simulink model "demapping"  (R2013a)
settings: Solver=VariableStepDiscrete  StartTime=0.0  StopTime=1  RelTol=1e-3
StopFcn:
  | figure(3)
  | hold off
  | plot([-1 1], [0 0],'k:');
  | hold on
  | plot([0 0], [-1 1],'k-');
  | plot([0 x_in_vec(1)], [0 y_in_vec(1)], 'r-','LineWidth',2);
  | plot([0 x_out_vec(1)], [0 y_out_vec(1)],'b-','LineWidth',2);
  | legend('X axis', 'Y axis', 'Input Vector','Output Vector',4);
  | xlabel('X');
  | ylabel('Y');
  | title('Input and Output Vectors');
  | axis([-1 1 -1 1]);
  | axis equal
libraries: xbsIndex_r4 x63
settings Model: Creator=lcrockett  LastModifiedBy=hebin
settings DataIOCC: SignalLoggingSaveFormat=ModelDataLogs
settings OptimizationCC: InlineParams=on  ExpressionDepthLimit=2147483647  InitFltsAndDblsToZero=on
settings DebuggingCC: SaveWithParameterizedLinksMsg=none  FcnCallInpInsideContextMsg=UseLocalSettings  StrictBusMsg=Warning
settings GRTTargetCC: TargetFcnLib=ansi_tfl_tmw.mat  CombineOutputUpdateFcns=off  GRTInterface=on

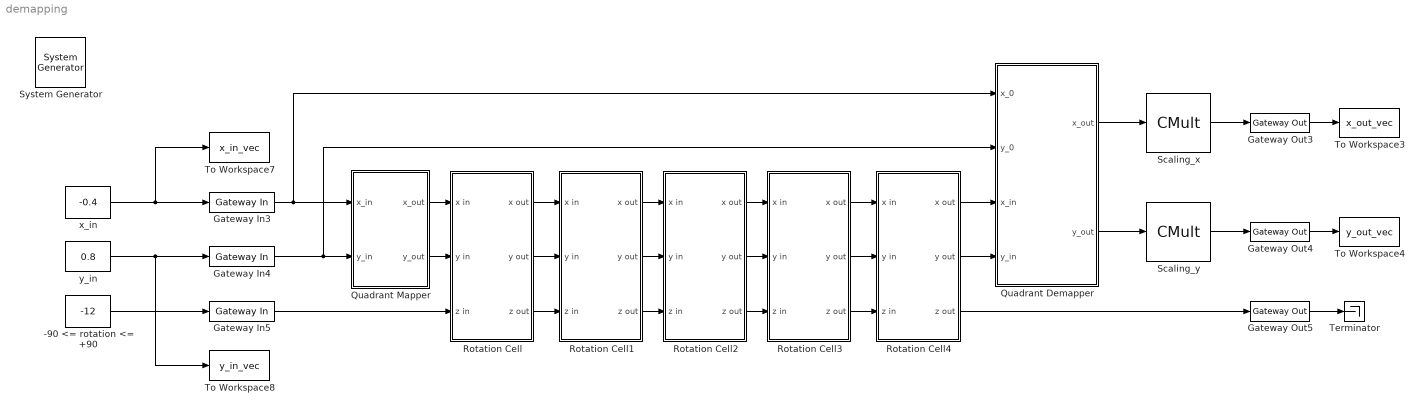
== system demapping ==
  " System Generator" : xbsIndex_r4/ System Generator  Tag=genX  xilinxfamily=virtex2p  part=xc2vp30  speed=-7  package=ff896  synthesis_tool=XST  clock_wrapper=Clock Enables  directory=./netlist  proj_type=Vivado  Synth_file=Vivado Synthesis Defaults  Impl_file=Vivado Implementation Defaults  testbench=off  simulink_period=1  sysclk_period=100  dcm_input_clock_period=100  incr_netlist=off  trim_vbits=Everywhere in SubSystem  dbl_ovrd=According to Block Masks  core_generation=According to Block Masks  run_coregen=off  deprecated_control=off  eval_field=0  block_type=sysgen
      settings: block_version=10.1.2
  -90 <= rotation <= +90 : Constant  Value=-12  SampleTime=1
  Gateway In3 : xbsIndex_r4/Gateway In  gui_display_data_type=Fixed-point  arith_type="Signed  (2's comp)"  n_bits=15  bin_pt=12  preci_type=Single  exp_width=8  frac_width=24  quantization="Round  (unbiased: +/- Inf)"  overflow=Saturate  period=1  UseAsADC=off  ADCChannel='1'  interface=None  automatic_assignment=on  address_offset=hex2dec('00')  intf_description=''  timing_constraint=None  locs_specified=off  LOCs={}  inherit_from_input=off  hdl_port=on  dbl_ovrd=off  io_standard={}  block_type=gatewayin
      settings: infoedit="Gateway in block.  Converts inputs of type Simulink integer, double and fixed point to  Xilinx fixed point type.<P><P>Hardware notes:  In hardware these blocks become top level input ports."  block_version=10.1.2
  Gateway In4 : xbsIndex_r4/Gateway In  gui_display_data_type=Fixed-point  arith_type="Signed  (2's comp)"  n_bits=15  bin_pt=12  preci_type=Single  exp_width=8  frac_width=24  quantization="Round  (unbiased: +/- Inf)"  overflow=Saturate  period=1  UseAsADC=off  ADCChannel='1'  interface=None  automatic_assignment=on  address_offset=hex2dec('00')  intf_description=''  timing_constraint=None  locs_specified=off  LOCs={}  inherit_from_input=off  hdl_port=on  dbl_ovrd=off  io_standard={}  block_type=gatewayin
      settings: infoedit="Gateway in block.  Converts inputs of type Simulink integer, double and fixed point to  Xilinx fixed point type.<P><P>Hardware notes:  In hardware these blocks become top level input ports."  block_version=10.1.2
  Gateway In5 : xbsIndex_r4/Gateway In  gui_display_data_type=Fixed-point  arith_type="Signed  (2's comp)"  n_bits=20  bin_pt=12  preci_type=Single  exp_width=8  frac_width=24  quantization="Round  (unbiased: +/- Inf)"  overflow=Saturate  period=1  UseAsADC=off  ADCChannel='1'  interface=None  automatic_assignment=on  address_offset=hex2dec('00')  intf_description=''  timing_constraint=None  locs_specified=off  LOCs={}  inherit_from_input=off  hdl_port=on  dbl_ovrd=off  io_standard={}  block_type=gatewayin
      settings: infoedit="Gateway in block.  Converts inputs of type Simulink integer, double and fixed point to  Xilinx fixed point type.<P><P>Hardware notes:  In hardware these blocks become top level input ports."  block_version=10.1.2
  Gateway Out3 : xbsIndex_r4/Gateway Out  inherit_from_input=off  hdl_port=on  rows=1  columns=1  UseAsDAC=off  DACChannel='1'  interface=None  automatic_assignment=on  address_offset=hex2dec('00')  intf_description=''  timing_constraint=None  locs_specified=off  LOCs={}  io_standard={}  block_type=gatewayout
      settings: infoedit="Gateway out block.  Converts Xilinx fixed point inputs into ouputs of type Simulink integer, double, or fixed point.<P><P>Hardware notes:  In hardware these blocks become top level output ports or are discarded, depending on how they are configured."  block_version=10.1.2
  Gateway Out4 : xbsIndex_r4/Gateway Out  inherit_from_input=off  hdl_port=on  rows=1  columns=1  UseAsDAC=off  DACChannel='1'  interface=None  automatic_assignment=on  address_offset=hex2dec('00')  intf_description=''  timing_constraint=None  locs_specified=off  LOCs={}  io_standard={}  block_type=gatewayout
      settings: infoedit="Gateway out block.  Converts Xilinx fixed point inputs into ouputs of type Simulink integer, double, or fixed point.<P><P>Hardware notes:  In hardware these blocks become top level output ports or are discarded, depending on how they are configured."  block_version=10.1.2
  Gateway Out5 : xbsIndex_r4/Gateway Out  inherit_from_input=off  hdl_port=on  rows=1  columns=1  UseAsDAC=off  DACChannel='1'  interface=None  automatic_assignment=on  address_offset=hex2dec('00')  intf_description=''  timing_constraint=None  locs_specified=off  LOCs={}  io_standard={}  block_type=gatewayout
      settings: infoedit="Gateway out block.  Converts Xilinx fixed point inputs into ouputs of type Simulink integer, double, or fixed point.<P><P>Hardware notes:  In hardware these blocks become top level output ports or are discarded, depending on how they are configured."  block_version=10.1.2
  Quadrant Demapper : Subsystem
  Quadrant Mapper : Subsystem
  Rotation Cell : Subsystem  mask(Rotation Cell){i=0}
      mask prompts: i "Number of Iterations (i)"
  Rotation Cell1 : Subsystem  mask(Rotation Cell){i=1}
      mask prompts: i "Number of Iterations (i)"
  Rotation Cell2 : Subsystem  mask(Rotation Cell){i=2}
      mask prompts: i "Number of Iterations (i)"
  Rotation Cell3 : Subsystem  mask(Rotation Cell){i=3}
      mask prompts: i "Number of Iterations (i)"
  Rotation Cell4 : Subsystem  mask(Rotation Cell){i=4}
      mask prompts: i "Number of Iterations (i)"
  Scaling_x : xbsIndex_r4/CMult  const=0.607648256256168  gui_display_data_type=Fixed-point  const_n_bits=15  const_bin_pt=12  float_type=Single  exp_bits=8  fraction_bits=24  en=off  latency=0  precision=User Defined  arith_type="Signed  (2's comp)"  n_bits=15  bin_pt=12  quantization=Truncate  overflow=Wrap  use_behavioral_HDL=off  mem_type=Distributed RAM  pipeline=off  use_rpm=off  placement_style=Rectangular Shape  dbl_ovrd=off  block_type=cmult
      settings: block_version=10.1.2
  Scaling_y : xbsIndex_r4/CMult  const=0.607648256256168  gui_display_data_type=Fixed-point  const_n_bits=15  const_bin_pt=12  float_type=Single  exp_bits=8  fraction_bits=24  en=off  latency=0  precision=User Defined  arith_type="Signed  (2's comp)"  n_bits=15  bin_pt=12  quantization=Truncate  overflow=Wrap  use_behavioral_HDL=off  mem_type=Distributed RAM  pipeline=off  use_rpm=off  placement_style=Rectangular Shape  dbl_ovrd=off  block_type=cmult
      settings: block_version=10.1.2
  Terminator : Terminator
  To Workspace3 : ToWorkspace  VariableName=x_out_vec  SampleTime=-1
  To Workspace4 : ToWorkspace  VariableName=y_out_vec  SampleTime=-1
  To Workspace7 : ToWorkspace  VariableName=x_in_vec  SampleTime=-1
  To Workspace8 : ToWorkspace  VariableName=y_in_vec  SampleTime=-1
  x_in : Constant  Value=-0.4  SampleTime=1
  y_in : Constant  Value=0.8  SampleTime=1
  wires:
  Gateway In5/1 -> Rotation Cell/3(z in)
  -90 <= rotation <= +90/1 -> Gateway In5/1
  x_in/1 -> Gateway In3/1, To Workspace7/1
  y_in/1 -> To Workspace8/1, Gateway In4/1
  Gateway Out3/1 -> To Workspace3/1
  Gateway Out4/1 -> To Workspace4/1
  Gateway Out5/1 -> Terminator/1
  Gateway In3/1 -> Quadrant Mapper/1(x_in), Quadrant Demapper/1(x_0)
  Quadrant Mapper/1(x_out) -> Rotation Cell/1(x in)
  Gateway In4/1 -> Quadrant Mapper/2(y_in), Quadrant Demapper/2(y_0)
  Quadrant Mapper/2(y_out) -> Rotation Cell/2(y in)
  Rotation Cell/1(x out) -> Rotation Cell1/1(x in)
  Rotation Cell/2(y out) -> Rotation Cell1/2(y in)
  Rotation Cell/3(z out) -> Rotation Cell1/3(z in)
  Rotation Cell1/1(x out) -> Rotation Cell2/1(x in)
  Rotation Cell1/2(y out) -> Rotation Cell2/2(y in)
  Rotation Cell1/3(z out) -> Rotation Cell2/3(z in)
  Rotation Cell2/1(x out) -> Rotation Cell3/1(x in)
  Rotation Cell2/2(y out) -> Rotation Cell3/2(y in)
  Rotation Cell2/3(z out) -> Rotation Cell3/3(z in)
  Rotation Cell3/1(x out) -> Rotation Cell4/1(x in)
  Rotation Cell3/2(y out) -> Rotation Cell4/2(y in)
  Rotation Cell3/3(z out) -> Rotation Cell4/3(z in)
  Scaling_x/1 -> Gateway Out3/1
  Rotation Cell4/3(z out) -> Gateway Out5/1
  Rotation Cell4/2(y out) -> Quadrant Demapper/4(y_in)
  Rotation Cell4/1(x out) -> Quadrant Demapper/3(x_in)
  Quadrant Demapper/1(x_out) -> Scaling_x/1
  Quadrant Demapper/2(y_out) -> Scaling_y/1
  Scaling_y/1 -> Gateway Out4/1

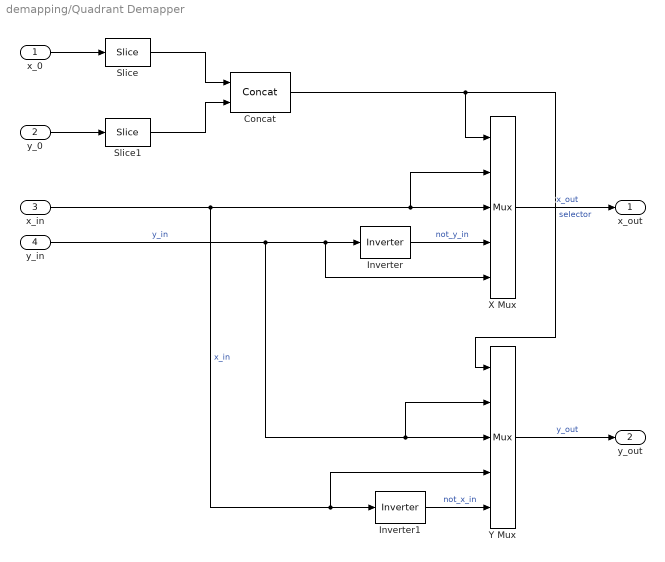
== system demapping/Quadrant Demapper ==
  x_0 : Inport
  y_0 : Inport  Port=2
  x_in : Inport  Port=3
  y_in : Inport  Port=4
  Concat : xbsIndex_r4/Concat  num_inputs=2  dbl_ovrd=off  block_type=concat
      settings: block_version=10.1.2
  Inverter : xbsIndex_r4/Inverter  en=off  latency=0  dbl_ovrd=off  block_type=inv
      settings: block_version=10.1.2
  Inverter1 : xbsIndex_r4/Inverter  en=off  latency=0  dbl_ovrd=off  block_type=inv
      settings: block_version=10.1.2
  Slice : xbsIndex_r4/Slice  nbits=1  boolean_output=on  mode=Upper Bit Location + Width  bit1=0  base1=MSB of Input  bit0=0  base0=LSB of Input  dbl_ovrd=off  block_type=slice
      settings: infoedit="Extracts a given range of bits from each input sample and presents it at the output.  The output type is ordinarily unsigned with binary point at zero, but can be Boolean when the slice is one bit wide.<P><P>Hardware notes: In hardware this block costs nothing."  block_version=VER_STRING_GOES_HERE
  Slice1 : xbsIndex_r4/Slice  nbits=1  boolean_output=on  mode=Upper Bit Location + Width  bit1=0  base1=MSB of Input  bit0=0  base0=LSB of Input  dbl_ovrd=off  block_type=slice
      settings: infoedit="Extracts a given range of bits from each input sample and presents it at the output.  The output type is ordinarily unsigned with binary point at zero, but can be Boolean when the slice is one bit wide.<P><P>Hardware notes: In hardware this block costs nothing."  block_version=VER_STRING_GOES_HERE
  X Mux : xbsIndex_r4/Mux  inputs=4  en=off  latency=0  precision=User Defined  arith_type="Signed  (2's comp)"  n_bits=16  bin_pt=14  quantization=Truncate  overflow=Wrap  dbl_ovrd=off  block_type=mux
      settings: xl_area=[0, 0, 0, 0, 0, 0, 0]  block_version=VER_STRING_GOES_HERE
  Y Mux : xbsIndex_r4/Mux  inputs=4  en=off  latency=0  precision=User Defined  arith_type="Signed  (2's comp)"  n_bits=16  bin_pt=14  quantization=Truncate  overflow=Wrap  dbl_ovrd=off  block_type=mux
      settings: xl_area=[0, 0, 0, 0, 0, 0, 0]  block_version=VER_STRING_GOES_HERE
  x_out : Outport
  y_out : Outport  Port=2
  wires:
  Slice/1 -> Concat/1
  Slice1/1 -> Concat/2
  Concat/1 -> X Mux/1, Y Mux/1  "selector"
  y_0/1 -> Slice1/1
  X Mux/1 -> x_out/1  "x_out"
  Y Mux/1 -> y_out/1  "y_out"
  x_0/1 -> Slice/1
  x_in/1 -> X Mux/2, X Mux/3, Inverter1/1, Y Mux/4  "x_in"
  y_in/1 -> X Mux/5, Inverter/1, Y Mux/3, Y Mux/2  "y_in"
  Inverter/1 -> X Mux/4  "not_y_in"
  Inverter1/1 -> Y Mux/5  "not_x_in"

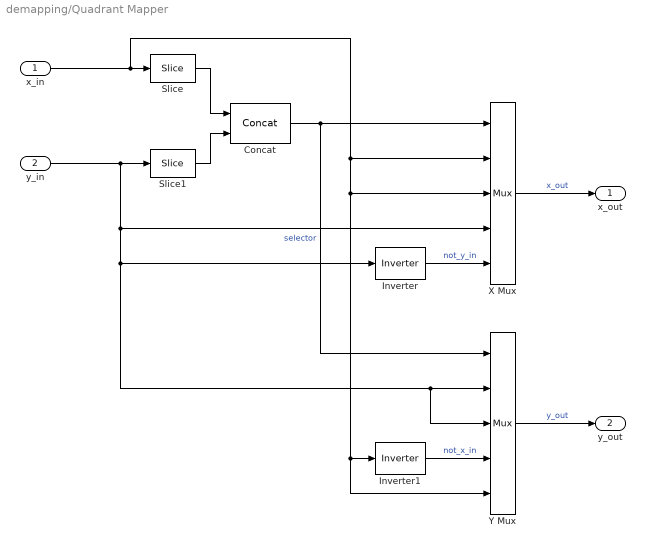
== system demapping/Quadrant Mapper ==
  x_in : Inport
  y_in : Inport  Port=2
  Concat : xbsIndex_r4/Concat  num_inputs=2  dbl_ovrd=off  block_type=concat
      settings: block_version=10.1.2
  Inverter : xbsIndex_r4/Inverter  en=off  latency=0  dbl_ovrd=off  block_type=inv
      settings: block_version=10.1.2
  Inverter1 : xbsIndex_r4/Inverter  en=off  latency=0  dbl_ovrd=off  block_type=inv
      settings: block_version=10.1.2
  Slice : xbsIndex_r4/Slice  nbits=1  boolean_output=on  mode=Upper Bit Location + Width  bit1=0  base1=MSB of Input  bit0=0  base0=LSB of Input  dbl_ovrd=off  block_type=slice
      settings: infoedit="Extracts a given range of bits from each input sample and presents it at the output.  The output type is ordinarily unsigned with binary point at zero, but can be Boolean when the slice is one bit wide.<P><P>Hardware notes: In hardware this block costs nothing."  block_version=VER_STRING_GOES_HERE
  Slice1 : xbsIndex_r4/Slice  nbits=1  boolean_output=on  mode=Upper Bit Location + Width  bit1=0  base1=MSB of Input  bit0=0  base0=LSB of Input  dbl_ovrd=off  block_type=slice
      settings: infoedit="Extracts a given range of bits from each input sample and presents it at the output.  The output type is ordinarily unsigned with binary point at zero, but can be Boolean when the slice is one bit wide.<P><P>Hardware notes: In hardware this block costs nothing."  block_version=VER_STRING_GOES_HERE
  X Mux : xbsIndex_r4/Mux  inputs=4  en=off  latency=0  precision=User Defined  arith_type="Signed  (2's comp)"  n_bits=16  bin_pt=14  quantization=Truncate  overflow=Wrap  dbl_ovrd=off  block_type=mux
      settings: xl_area=[0, 0, 0, 0, 0, 0, 0]  block_version=VER_STRING_GOES_HERE
  Y Mux : xbsIndex_r4/Mux  inputs=4  en=off  latency=0  precision=User Defined  arith_type="Signed  (2's comp)"  n_bits=16  bin_pt=14  quantization=Truncate  overflow=Wrap  dbl_ovrd=off  block_type=mux
      settings: xl_area=[0, 0, 0, 0, 0, 0, 0]  block_version=VER_STRING_GOES_HERE
  x_out : Outport
  y_out : Outport  Port=2
  wires:
  Slice/1 -> Concat/1
  Slice1/1 -> Concat/2
  Concat/1 -> X Mux/1, Y Mux/1  "selector"
  Inverter/1 -> X Mux/5  "not_y_in"
  Inverter1/1 -> Y Mux/4  "not_x_in"
  x_in/1 -> Slice/1, X Mux/2, X Mux/3, Y Mux/5, Inverter1/1
  y_in/1 -> Slice1/1, X Mux/4, Inverter/1, Y Mux/2, Y Mux/3
  X Mux/1 -> x_out/1  "x_out"
  Y Mux/1 -> y_out/1  "y_out"

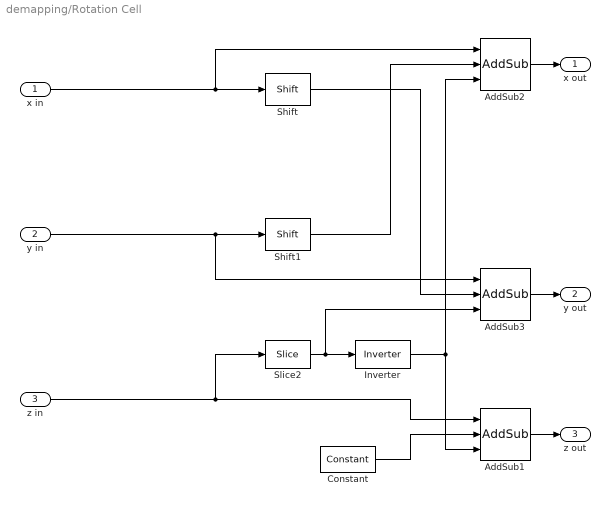
== system demapping/Rotation Cell ==
  x in : Inport
  y in : Inport  Port=2
  z in : Inport  Port=3
  AddSub1 : xbsIndex_r4/AddSub  mode=Addition or Subtraction  use_carryin=off  use_carryout=off  en=off  latency=0  precision=User Defined  arith_type="Signed  (2's comp)"  n_bits=20  bin_pt=12  quantization=Truncate  overflow=Wrap  dbl_ovrd=off  use_behavioral_HDL=on  pipelined=off  use_rpm=on  block_type=addsub
      settings: xl_area=[0, 0, 0, 0, 0, 0, 0]  block_version=VER_STRING_GOES_HERE
  AddSub2 : xbsIndex_r4/AddSub  mode=Addition or Subtraction  use_carryin=off  use_carryout=off  en=off  latency=0  precision=User Defined  arith_type="Signed  (2's comp)"  n_bits=15  bin_pt=12  quantization=Truncate  overflow=Wrap  dbl_ovrd=off  use_behavioral_HDL=on  pipelined=off  use_rpm=on  block_type=addsub
      settings: xl_area=[0, 0, 0, 0, 0, 0, 0]  block_version=VER_STRING_GOES_HERE
  AddSub3 : xbsIndex_r4/AddSub  mode=Addition or Subtraction  use_carryin=off  use_carryout=off  en=off  latency=0  precision=User Defined  arith_type="Signed  (2's comp)"  n_bits=15  bin_pt=12  quantization=Truncate  overflow=Wrap  dbl_ovrd=off  use_behavioral_HDL=on  pipelined=off  use_rpm=on  block_type=addsub
      settings: xl_area=[0, 0, 0, 0, 0, 0, 0]  block_version=VER_STRING_GOES_HERE
  Constant : xbsIndex_r4/Constant  arith_type=Signed (2's comp)  const=atand(2^-i)  n_bits=20  bin_pt=12  explicit_period=off  period=1  equ=P=C  opselect=C  inp2=PCIN>>17  opr=+  inp1=P  carry=CIN  dbl_ovrd=off  block_type=constant
      settings: block_version=10.1.2
  Inverter : xbsIndex_r4/Inverter  en=off  latency=0  dbl_ovrd=off  block_type=inv
      settings: block_version=10.1.2
  Shift : xbsIndex_r4/Shift  shift_dir=Right  shift_bits=i  en=off  latency=0  precision=User Defined  arith_type="Signed  (2's comp)"  n_bits=15  bin_pt=12  quantization=Truncate  overflow=Wrap  dbl_ovrd=off  block_type=shift
      settings: xl_area=[0, 0, 0, 0, 0, 0, 0]  block_version=VER_STRING_GOES_HERE
  Shift1 : xbsIndex_r4/Shift  shift_dir=Right  shift_bits=i  en=off  latency=0  precision=User Defined  arith_type="Signed  (2's comp)"  n_bits=15  bin_pt=12  quantization=Truncate  overflow=Wrap  dbl_ovrd=off  block_type=shift
      settings: xl_area=[0, 0, 0, 0, 0, 0, 0]  block_version=VER_STRING_GOES_HERE
  Slice2 : xbsIndex_r4/Slice  nbits=1  boolean_output=on  mode=Upper Bit Location + Width  bit1=0  base1=MSB of Input  bit0=0  base0=LSB of Input  dbl_ovrd=off  block_type=slice
      settings: infoedit="Extracts a given range of bits from each input sample and presents it at the output.  The output type is ordinarily unsigned with binary point at zero, but can be Boolean when the slice is one bit wide.<P><P>Hardware notes: In hardware this block costs nothing."  block_version=VER_STRING_GOES_HERE
  x out : Outport
  y out : Outport  Port=2
  z out : Outport  Port=3
  wires:
  x in/1 -> AddSub2/1, Shift/1
  y in/1 -> AddSub3/1, Shift1/1
  Shift1/1 -> AddSub2/2
  Shift/1 -> AddSub3/2
  AddSub2/1 -> x out/1
  AddSub3/1 -> y out/1
  z in/1 -> AddSub1/1, Slice2/1
  Constant/1 -> AddSub1/2
  Slice2/1 -> Inverter/1, AddSub3/3
  AddSub1/1 -> z out/1
  Inverter/1 -> AddSub1/3, AddSub2/3

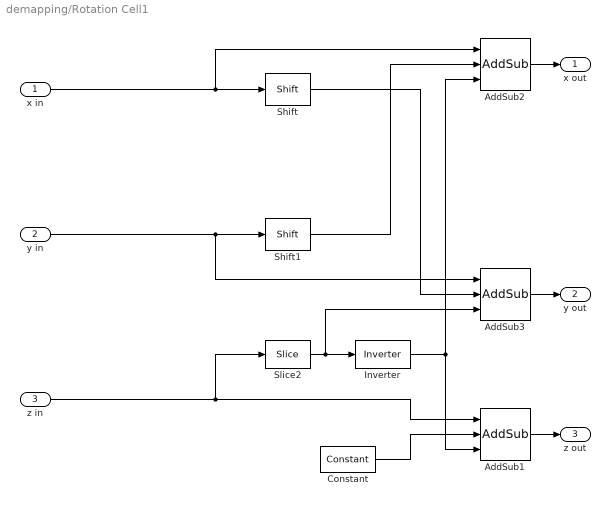
== system demapping/Rotation Cell1 ==
  x in : Inport
  y in : Inport  Port=2
  z in : Inport  Port=3
  AddSub1 : xbsIndex_r4/AddSub  mode=Addition or Subtraction  use_carryin=off  use_carryout=off  en=off  latency=0  precision=User Defined  arith_type="Signed  (2's comp)"  n_bits=20  bin_pt=12  quantization=Truncate  overflow=Wrap  dbl_ovrd=off  use_behavioral_HDL=on  pipelined=off  use_rpm=on  block_type=addsub
      settings: xl_area=[0, 0, 0, 0, 0, 0, 0]  block_version=VER_STRING_GOES_HERE
  AddSub2 : xbsIndex_r4/AddSub  mode=Addition or Subtraction  use_carryin=off  use_carryout=off  en=off  latency=0  precision=User Defined  arith_type="Signed  (2's comp)"  n_bits=15  bin_pt=12  quantization=Truncate  overflow=Wrap  dbl_ovrd=off  use_behavioral_HDL=on  pipelined=off  use_rpm=on  block_type=addsub
      settings: xl_area=[0, 0, 0, 0, 0, 0, 0]  block_version=VER_STRING_GOES_HERE
  AddSub3 : xbsIndex_r4/AddSub  mode=Addition or Subtraction  use_carryin=off  use_carryout=off  en=off  latency=0  precision=User Defined  arith_type="Signed  (2's comp)"  n_bits=15  bin_pt=12  quantization=Truncate  overflow=Wrap  dbl_ovrd=off  use_behavioral_HDL=on  pipelined=off  use_rpm=on  block_type=addsub
      settings: xl_area=[0, 0, 0, 0, 0, 0, 0]  block_version=VER_STRING_GOES_HERE
  Constant : xbsIndex_r4/Constant  arith_type=Signed (2's comp)  const=atand(2^-i)  n_bits=20  bin_pt=12  explicit_period=off  period=1  equ=P=C  opselect=C  inp2=PCIN>>17  opr=+  inp1=P  carry=CIN  dbl_ovrd=off  block_type=constant
      settings: block_version=10.1.2
  Inverter : xbsIndex_r4/Inverter  en=off  latency=0  dbl_ovrd=off  block_type=inv
      settings: block_version=10.1.2
  Shift : xbsIndex_r4/Shift  shift_dir=Right  shift_bits=i  en=off  latency=0  precision=User Defined  arith_type="Signed  (2's comp)"  n_bits=15  bin_pt=12  quantization=Truncate  overflow=Wrap  dbl_ovrd=off  block_type=shift
      settings: xl_area=[0, 0, 0, 0, 0, 0, 0]  block_version=VER_STRING_GOES_HERE
  Shift1 : xbsIndex_r4/Shift  shift_dir=Right  shift_bits=i  en=off  latency=0  precision=User Defined  arith_type="Signed  (2's comp)"  n_bits=15  bin_pt=12  quantization=Truncate  overflow=Wrap  dbl_ovrd=off  block_type=shift
      settings: xl_area=[0, 0, 0, 0, 0, 0, 0]  block_version=VER_STRING_GOES_HERE
  Slice2 : xbsIndex_r4/Slice  nbits=1  boolean_output=on  mode=Upper Bit Location + Width  bit1=0  base1=MSB of Input  bit0=0  base0=LSB of Input  dbl_ovrd=off  block_type=slice
      settings: infoedit="Extracts a given range of bits from each input sample and presents it at the output.  The output type is ordinarily unsigned with binary point at zero, but can be Boolean when the slice is one bit wide.<P><P>Hardware notes: In hardware this block costs nothing."  block_version=VER_STRING_GOES_HERE
  x out : Outport
  y out : Outport  Port=2
  z out : Outport  Port=3
  wires:
  x in/1 -> AddSub2/1, Shift/1
  y in/1 -> AddSub3/1, Shift1/1
  Shift1/1 -> AddSub2/2
  Shift/1 -> AddSub3/2
  AddSub2/1 -> x out/1
  AddSub3/1 -> y out/1
  z in/1 -> AddSub1/1, Slice2/1
  Constant/1 -> AddSub1/2
  Slice2/1 -> Inverter/1, AddSub3/3
  AddSub1/1 -> z out/1
  Inverter/1 -> AddSub1/3, AddSub2/3

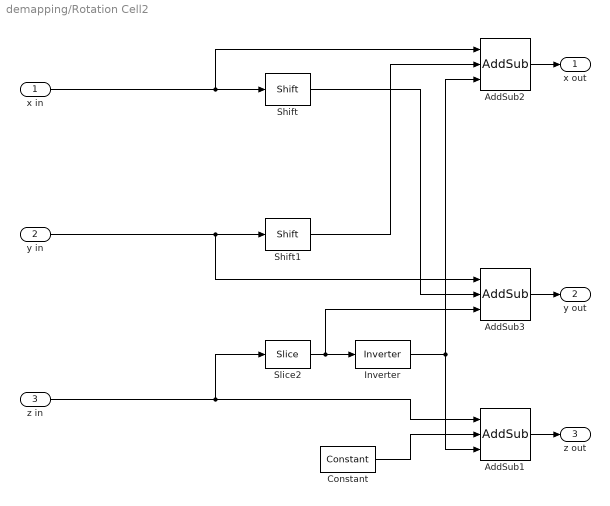
== system demapping/Rotation Cell2 ==
  x in : Inport
  y in : Inport  Port=2
  z in : Inport  Port=3
  AddSub1 : xbsIndex_r4/AddSub  mode=Addition or Subtraction  use_carryin=off  use_carryout=off  en=off  latency=0  precision=User Defined  arith_type="Signed  (2's comp)"  n_bits=20  bin_pt=12  quantization=Truncate  overflow=Wrap  dbl_ovrd=off  use_behavioral_HDL=on  pipelined=off  use_rpm=on  block_type=addsub
      settings: xl_area=[0, 0, 0, 0, 0, 0, 0]  block_version=VER_STRING_GOES_HERE
  AddSub2 : xbsIndex_r4/AddSub  mode=Addition or Subtraction  use_carryin=off  use_carryout=off  en=off  latency=0  precision=User Defined  arith_type="Signed  (2's comp)"  n_bits=15  bin_pt=12  quantization=Truncate  overflow=Wrap  dbl_ovrd=off  use_behavioral_HDL=on  pipelined=off  use_rpm=on  block_type=addsub
      settings: xl_area=[0, 0, 0, 0, 0, 0, 0]  block_version=VER_STRING_GOES_HERE
  AddSub3 : xbsIndex_r4/AddSub  mode=Addition or Subtraction  use_carryin=off  use_carryout=off  en=off  latency=0  precision=User Defined  arith_type="Signed  (2's comp)"  n_bits=15  bin_pt=12  quantization=Truncate  overflow=Wrap  dbl_ovrd=off  use_behavioral_HDL=on  pipelined=off  use_rpm=on  block_type=addsub
      settings: xl_area=[0, 0, 0, 0, 0, 0, 0]  block_version=VER_STRING_GOES_HERE
  Constant : xbsIndex_r4/Constant  arith_type=Signed (2's comp)  const=atand(2^-i)  n_bits=20  bin_pt=12  explicit_period=off  period=1  equ=P=C  opselect=C  inp2=PCIN>>17  opr=+  inp1=P  carry=CIN  dbl_ovrd=off  block_type=constant
      settings: block_version=10.1.2
  Inverter : xbsIndex_r4/Inverter  en=off  latency=0  dbl_ovrd=off  block_type=inv
      settings: block_version=10.1.2
  Shift : xbsIndex_r4/Shift  shift_dir=Right  shift_bits=i  en=off  latency=0  precision=User Defined  arith_type="Signed  (2's comp)"  n_bits=15  bin_pt=12  quantization=Truncate  overflow=Wrap  dbl_ovrd=off  block_type=shift
      settings: xl_area=[0, 0, 0, 0, 0, 0, 0]  block_version=VER_STRING_GOES_HERE
  Shift1 : xbsIndex_r4/Shift  shift_dir=Right  shift_bits=i  en=off  latency=0  precision=User Defined  arith_type="Signed  (2's comp)"  n_bits=15  bin_pt=12  quantization=Truncate  overflow=Wrap  dbl_ovrd=off  block_type=shift
      settings: xl_area=[0, 0, 0, 0, 0, 0, 0]  block_version=VER_STRING_GOES_HERE
  Slice2 : xbsIndex_r4/Slice  nbits=1  boolean_output=on  mode=Upper Bit Location + Width  bit1=0  base1=MSB of Input  bit0=0  base0=LSB of Input  dbl_ovrd=off  block_type=slice
      settings: infoedit="Extracts a given range of bits from each input sample and presents it at the output.  The output type is ordinarily unsigned with binary point at zero, but can be Boolean when the slice is one bit wide.<P><P>Hardware notes: In hardware this block costs nothing."  block_version=VER_STRING_GOES_HERE
  x out : Outport
  y out : Outport  Port=2
  z out : Outport  Port=3
  wires:
  x in/1 -> AddSub2/1, Shift/1
  y in/1 -> AddSub3/1, Shift1/1
  Shift1/1 -> AddSub2/2
  Shift/1 -> AddSub3/2
  AddSub2/1 -> x out/1
  AddSub3/1 -> y out/1
  z in/1 -> AddSub1/1, Slice2/1
  Constant/1 -> AddSub1/2
  Slice2/1 -> Inverter/1, AddSub3/3
  AddSub1/1 -> z out/1
  Inverter/1 -> AddSub1/3, AddSub2/3

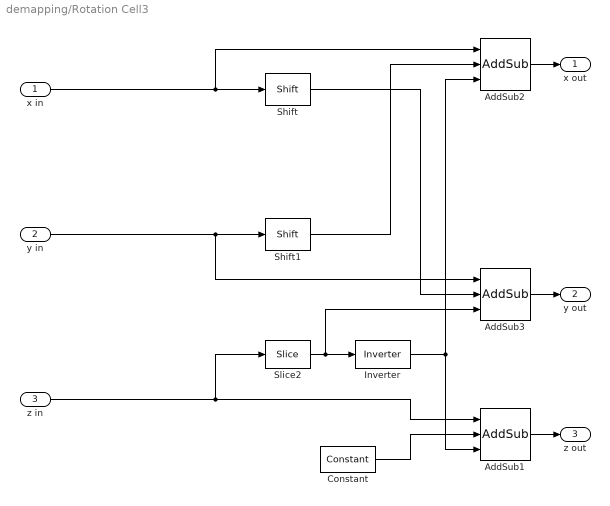
== system demapping/Rotation Cell3 ==
  x in : Inport
  y in : Inport  Port=2
  z in : Inport  Port=3
  AddSub1 : xbsIndex_r4/AddSub  mode=Addition or Subtraction  use_carryin=off  use_carryout=off  en=off  latency=0  precision=User Defined  arith_type="Signed  (2's comp)"  n_bits=20  bin_pt=12  quantization=Truncate  overflow=Wrap  dbl_ovrd=off  use_behavioral_HDL=on  pipelined=off  use_rpm=on  block_type=addsub
      settings: xl_area=[0, 0, 0, 0, 0, 0, 0]  block_version=VER_STRING_GOES_HERE
  AddSub2 : xbsIndex_r4/AddSub  mode=Addition or Subtraction  use_carryin=off  use_carryout=off  en=off  latency=0  precision=User Defined  arith_type="Signed  (2's comp)"  n_bits=15  bin_pt=12  quantization=Truncate  overflow=Wrap  dbl_ovrd=off  use_behavioral_HDL=on  pipelined=off  use_rpm=on  block_type=addsub
      settings: xl_area=[0, 0, 0, 0, 0, 0, 0]  block_version=VER_STRING_GOES_HERE
  AddSub3 : xbsIndex_r4/AddSub  mode=Addition or Subtraction  use_carryin=off  use_carryout=off  en=off  latency=0  precision=User Defined  arith_type="Signed  (2's comp)"  n_bits=15  bin_pt=12  quantization=Truncate  overflow=Wrap  dbl_ovrd=off  use_behavioral_HDL=on  pipelined=off  use_rpm=on  block_type=addsub
      settings: xl_area=[0, 0, 0, 0, 0, 0, 0]  block_version=VER_STRING_GOES_HERE
  Constant : xbsIndex_r4/Constant  arith_type=Signed (2's comp)  const=atand(2^-i)  n_bits=20  bin_pt=12  explicit_period=off  period=1  equ=P=C  opselect=C  inp2=PCIN>>17  opr=+  inp1=P  carry=CIN  dbl_ovrd=off  block_type=constant
      settings: block_version=10.1.2
  Inverter : xbsIndex_r4/Inverter  en=off  latency=0  dbl_ovrd=off  block_type=inv
      settings: block_version=10.1.2
  Shift : xbsIndex_r4/Shift  shift_dir=Right  shift_bits=i  en=off  latency=0  precision=User Defined  arith_type="Signed  (2's comp)"  n_bits=15  bin_pt=12  quantization=Truncate  overflow=Wrap  dbl_ovrd=off  block_type=shift
      settings: xl_area=[0, 0, 0, 0, 0, 0, 0]  block_version=VER_STRING_GOES_HERE
  Shift1 : xbsIndex_r4/Shift  shift_dir=Right  shift_bits=i  en=off  latency=0  precision=User Defined  arith_type="Signed  (2's comp)"  n_bits=15  bin_pt=12  quantization=Truncate  overflow=Wrap  dbl_ovrd=off  block_type=shift
      settings: xl_area=[0, 0, 0, 0, 0, 0, 0]  block_version=VER_STRING_GOES_HERE
  Slice2 : xbsIndex_r4/Slice  nbits=1  boolean_output=on  mode=Upper Bit Location + Width  bit1=0  base1=MSB of Input  bit0=0  base0=LSB of Input  dbl_ovrd=off  block_type=slice
      settings: infoedit="Extracts a given range of bits from each input sample and presents it at the output.  The output type is ordinarily unsigned with binary point at zero, but can be Boolean when the slice is one bit wide.<P><P>Hardware notes: In hardware this block costs nothing."  block_version=VER_STRING_GOES_HERE
  x out : Outport
  y out : Outport  Port=2
  z out : Outport  Port=3
  wires:
  x in/1 -> AddSub2/1, Shift/1
  y in/1 -> AddSub3/1, Shift1/1
  Shift1/1 -> AddSub2/2
  Shift/1 -> AddSub3/2
  AddSub2/1 -> x out/1
  AddSub3/1 -> y out/1
  z in/1 -> AddSub1/1, Slice2/1
  Constant/1 -> AddSub1/2
  Slice2/1 -> Inverter/1, AddSub3/3
  AddSub1/1 -> z out/1
  Inverter/1 -> AddSub1/3, AddSub2/3

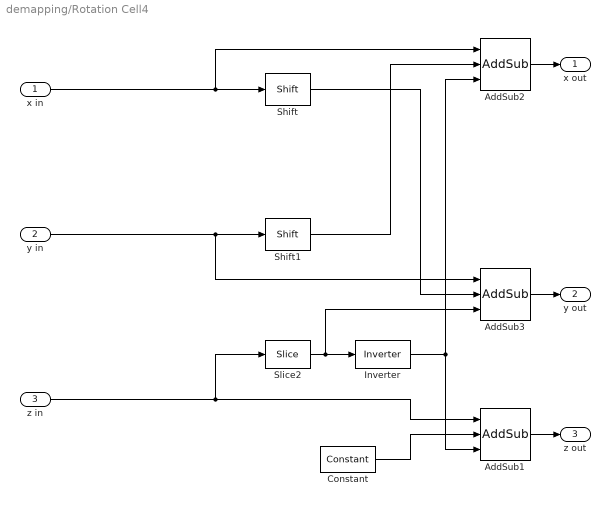
== system demapping/Rotation Cell4 ==
  x in : Inport
  y in : Inport  Port=2
  z in : Inport  Port=3
  AddSub1 : xbsIndex_r4/AddSub  mode=Addition or Subtraction  use_carryin=off  use_carryout=off  en=off  latency=0  precision=User Defined  arith_type="Signed  (2's comp)"  n_bits=20  bin_pt=12  quantization=Truncate  overflow=Wrap  dbl_ovrd=off  use_behavioral_HDL=on  pipelined=off  use_rpm=on  block_type=addsub
      settings: xl_area=[0, 0, 0, 0, 0, 0, 0]  block_version=VER_STRING_GOES_HERE
  AddSub2 : xbsIndex_r4/AddSub  mode=Addition or Subtraction  use_carryin=off  use_carryout=off  en=off  latency=0  precision=User Defined  arith_type="Signed  (2's comp)"  n_bits=15  bin_pt=12  quantization=Truncate  overflow=Wrap  dbl_ovrd=off  use_behavioral_HDL=on  pipelined=off  use_rpm=on  block_type=addsub
      settings: xl_area=[0, 0, 0, 0, 0, 0, 0]  block_version=VER_STRING_GOES_HERE
  AddSub3 : xbsIndex_r4/AddSub  mode=Addition or Subtraction  use_carryin=off  use_carryout=off  en=off  latency=0  precision=User Defined  arith_type="Signed  (2's comp)"  n_bits=15  bin_pt=12  quantization=Truncate  overflow=Wrap  dbl_ovrd=off  use_behavioral_HDL=on  pipelined=off  use_rpm=on  block_type=addsub
      settings: xl_area=[0, 0, 0, 0, 0, 0, 0]  block_version=VER_STRING_GOES_HERE
  Constant : xbsIndex_r4/Constant  arith_type=Signed (2's comp)  const=atand(2^-i)  n_bits=20  bin_pt=12  explicit_period=off  period=1  equ=P=C  opselect=C  inp2=PCIN>>17  opr=+  inp1=P  carry=CIN  dbl_ovrd=off  block_type=constant
      settings: block_version=10.1.2
  Inverter : xbsIndex_r4/Inverter  en=off  latency=0  dbl_ovrd=off  block_type=inv
      settings: block_version=10.1.2
  Shift : xbsIndex_r4/Shift  shift_dir=Right  shift_bits=i  en=off  latency=0  precision=User Defined  arith_type="Signed  (2's comp)"  n_bits=15  bin_pt=12  quantization=Truncate  overflow=Wrap  dbl_ovrd=off  block_type=shift
      settings: xl_area=[0, 0, 0, 0, 0, 0, 0]  block_version=VER_STRING_GOES_HERE
  Shift1 : xbsIndex_r4/Shift  shift_dir=Right  shift_bits=i  en=off  latency=0  precision=User Defined  arith_type="Signed  (2's comp)"  n_bits=15  bin_pt=12  quantization=Truncate  overflow=Wrap  dbl_ovrd=off  block_type=shift
      settings: xl_area=[0, 0, 0, 0, 0, 0, 0]  block_version=VER_STRING_GOES_HERE
  Slice2 : xbsIndex_r4/Slice  nbits=1  boolean_output=on  mode=Upper Bit Location + Width  bit1=0  base1=MSB of Input  bit0=0  base0=LSB of Input  dbl_ovrd=off  block_type=slice
      settings: infoedit="Extracts a given range of bits from each input sample and presents it at the output.  The output type is ordinarily unsigned with binary point at zero, but can be Boolean when the slice is one bit wide.<P><P>Hardware notes: In hardware this block costs nothing."  block_version=VER_STRING_GOES_HERE
  x out : Outport
  y out : Outport  Port=2
  z out : Outport  Port=3
  wires:
  x in/1 -> AddSub2/1, Shift/1
  y in/1 -> AddSub3/1, Shift1/1
  Shift1/1 -> AddSub2/2
  Shift/1 -> AddSub3/2
  AddSub2/1 -> x out/1
  AddSub3/1 -> y out/1
  z in/1 -> AddSub1/1, Slice2/1
  Constant/1 -> AddSub1/2
  Slice2/1 -> Inverter/1, AddSub3/3
  AddSub1/1 -> z out/1
  Inverter/1 -> AddSub1/3, AddSub2/3
